simulink model "InputANDOutput"  (R2020a)
settings: Solver=ode45  StartTime=0.0  StopTime=inf  RelTol=1e-3
model workspace (MAT data in the model file):
  f_air = [0 0 0 0 0 0 0 0 0 0 0 0 ... (1600 elements, 40x40)]
  f_co = [0 0 0 0 0 0 0 0 0 0 0 0 ... (1600 elements, 40x40)]
  f_co2 = [0 0 0 0 0 0 0 0 0 0 0 0 ... (1600 elements, 40x40)]
  f_eff = [268.575244449 268.264872911 267.869436682 267.479641954 267.095762268 266.718061676 266.346789136 265.982171792 265.624407005 265.273653012 264.930018082 264.5935481 ... (1600 elements, 40x40)]
  f_fuel = [0 0 0 0 0 0 0 0 0 0 0 0 ... (1600 elements, 40x40)]
  f_hc = [0 0 0 0 0 0 0 0 0 0 0 0 ... (1600 elements, 40x40)]
  f_nox = [0 0 0 0 0 0 0 0 0 0 0 0 ... (1600 elements, 40x40)]
  f_pm = [0 0 0 0 0 0 0 0 0 0 0 0 ... (1600 elements, 40x40)]
  f_tbrake = [0 1.249866 2.86153531579 4.47320463158 5 5 5 5 5 5 5 5 ... (1600 elements, 40x40)]
  f_tbrake_n_bpt = [0; 5000; 5184.21052632; 5368.42105263; 5552.63157895; 5736.84210526; 5921.05263158; 6105.26315789; 6289.47368421; 6473.68421053; 6657.89473684; 6842.10526316; 7026.31578947; 7210.52631579; 7394.73684211; 7578.94736842; 7763.15789474; 7947.36842105; 8131.57894737; 8315.78947368; 8500; 8684.21052632; 8868.42105263; 9052.63157895; 9236.84210526; 9421.05263158; 9605.26315789; 9789.47368421; 9973.68421053; 10157.8947368; 10342.1052632; 10526.3157895; 10710.5263158; 10894.7368421; 11078.9473684; 11263.1578947; 11447.3684211; 11631.5789474; 11815.7894737; 12000]
  f_tbrake_t_bpt = [0; 1.249866; 2.86153531579; 4.47320463158; 6.08487394737; 7.69654326316; 9.30821257895; 10.9198818947; 12.5315512105; 14.1432205263; 15.7548898421; 17.3665591579; 18.9782284737; 20.5898977895; 22.2015671053; 23.8132364211; 25.4249057368; 27.0365750526; 28.6482443684; 30.2599136842; 31.871583; 33.4832523158; 35.0949216316; 36.7065909474; 38.3182602632; 39.9299295789; 41.5415988947; 43.1532682105; 44.7649375263; 46.3766068421; 47.9882761579; 49.5999454737; 51.2116147895; 52.8232841053; 54.4349534211; 56.0466227368; 57.6582920526; 59.2699613684; 60.8816306842; 62.4933]
  f_texh = [627.001831863 630.861919966 635.838470358 640.813862919 645.787996701 650.760794403 655.732210496 660.7022409 665.670934417 670.638406034 675.604852198 680.570568039 ... (1600 elements, 40x40)]
undefined symbols (not defined in the file): maxtrq
libraries: autolibengctrlr x1, autolibsharedmappedengines x1
(part 1 of 3)
settings Model: DataDictionary=Data_diction.sldd  OrderedModelArguments=off  Creator=ASD  LastModifiedBy=44689
settings SolverCC: AlgebraicLoopSolver=LineSearch

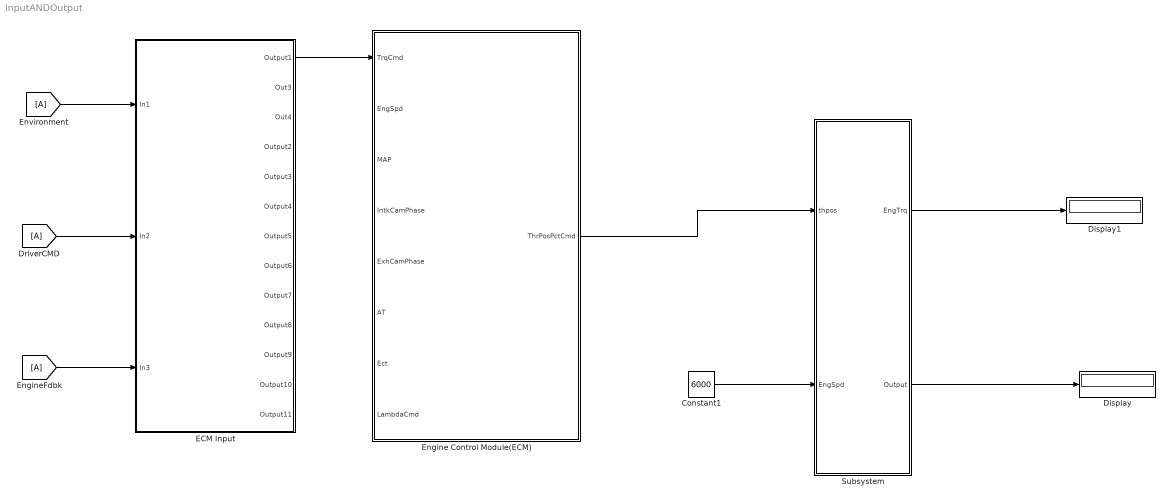
== system InputANDOutput ==
  Constant1 : Constant  Value=6000
  Display : Display
  Display1 : Display
  ECM Input : Subsystem
  Engine Control Module(ECM) : Subsystem
  Subsystem : Subsystem
  wires:
  Subsystem/1(EngTrq) -> Display1/1
  Engine Control Module(ECM)/1(ThrPosPctCmd) -> Subsystem/1(thpos)
  Subsystem/2(Output) -> Display/1
  Constant1/1 -> Subsystem/2(EngSpd)
  [A] -> ECM Input/1(In1)
  [A] -> ECM Input/2(In2)
  [A] -> ECM Input/3(In3)
  ECM Input/1(Output1) -> Engine Control Module(ECM)/1(TrqCmd)
